simulink model "SS_angulo_pos_planta_CLOSELOOP_simulink"  (R2023b)
settings: Solver=VariableStepAuto  StartTime=0.0  StopTime=15  RelTol=1e-6
values from neighbouring files (symbols this model uses):
  Planta = ss([0 0 1 0;0 0 0 1;0 0 -11.48 0;0 -35.39 0 -0.01639],[0;-0.3736;0.2846;-0.8948],[1 0 0 0;0 1 0 0],0)    [Script_generador.m]
undefined symbols (not defined in the file or in its folder): SS_An, SS_Po
settings Model: Creator=natih  LastModifiedBy=jmarin

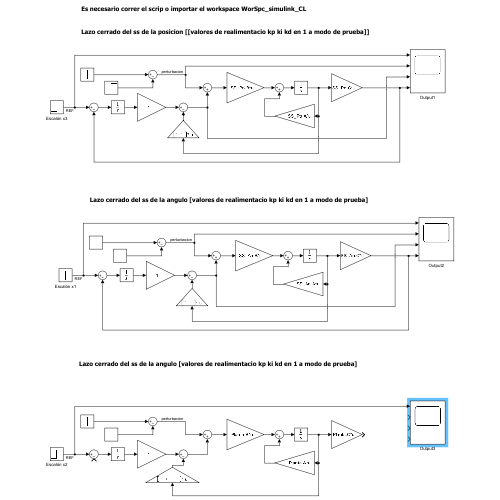
[thumbnail: Simulink's stored preview of the top-level diagram]
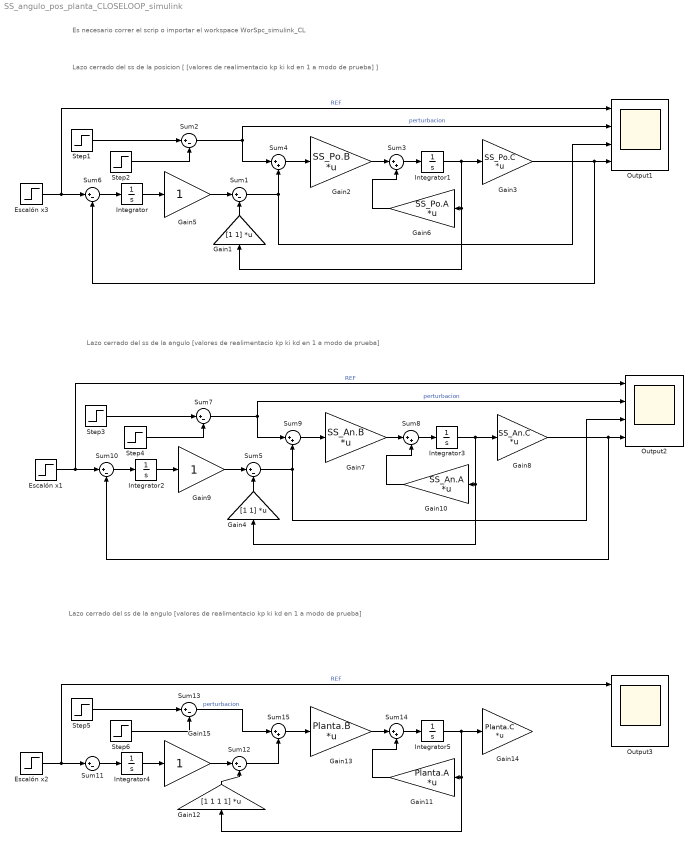
== system SS_angulo_pos_planta_CLOSELOOP_simulink ==
  note: Lazo cerrado del ss de la posicion [ [valores de realimentacio kp ki kd en 1 a modo de prueba] ]
  note: Lazo cerrado del ss de la angulo [valores de realimentacio kp ki kd en 1 a modo de prueba]
  note: Es necesario correr el scrip o importar el workspace WorSpc_simulink_CL
  note: Lazo cerrado del ss de la angulo [valores de realimentacio kp ki kd en 1 a modo de prueba]
  Escalón x1 : Step  Time=0.5  SampleTime=0
  Escalón x2 : Step  Time=0.5  SampleTime=0
  Escalón x3 : Step  Time=0.5  SampleTime=0
  Gain1 : Gain  Gain=[1 1]  Multiplication=Matrix(K*u)
  Gain10 : Gain  Gain=SS_An.A  Multiplication=Matrix(K*u)
  Gain11 : Gain  Gain=Planta.A  Multiplication=Matrix(K*u)
  Gain12 : Gain  Gain=[1 1 1 1]  Multiplication=Matrix(K*u)
  Gain13 : Gain  Gain=Planta.B  Multiplication=Matrix(K*u)
  Gain14 : Gain  Gain=Planta.C  Multiplication=Matrix(K*u)
  Gain15 : Gain
  Gain2 : Gain  Gain=SS_Po.B  Multiplication=Matrix(K*u)
  Gain3 : Gain  Gain=SS_Po.C  Multiplication=Matrix(K*u)
  Gain4 : Gain  Gain=[1 1]  Multiplication=Matrix(K*u)
  Gain5 : Gain
  Gain6 : Gain  Gain=SS_Po.A  Multiplication=Matrix(K*u)
  Gain7 : Gain  Gain=SS_An.B  Multiplication=Matrix(K*u)
  Gain8 : Gain  Gain=SS_An.C  Multiplication=Matrix(K*u)
  Gain9 : Gain
  Integrator{,1..5} (6 alike) : Integrator
  Output1 : Scope  NumInputPorts=4
  Output2 : Scope  NumInputPorts=4
  Output3 : Scope  NumInputPorts=4
  Step1 : Step  Time=6  After=0.3  SampleTime=0
  Step2 : Step  Time=11  After=0.3  SampleTime=0
  Step3 : Step  Time=6  After=0.3  SampleTime=0
  Step4 : Step  Time=11  After=0.3  SampleTime=0
  Step5 : Step  Time=6  After=0.3  SampleTime=0
  Step6 : Step  Time=11  After=0.3  SampleTime=0
  Sum{1..2,5..7,10..13} (9 alike) : Sum  Inputs=|+-
  Sum{3..4,8..9,14..15} (6 alike) : Sum  Inputs=|++
  wires:
  Step1/1 -> Sum2/1
  Escalón x3/1 -> Output1/1, Sum6/1  "REF"
  Step2/1 -> Sum2/2
  Sum6/1 -> Integrator/1
  Integrator/1 -> Gain5/1
  Gain5/1 -> Sum1/1
  Gain2/1 -> Sum3/1
  Sum3/1 -> Integrator1/1
  Integrator1/1 -> Gain1/1, Gain6/1, Gain3/1
  Gain3/1 -> Sum6/2, Output1/4
  Gain1/1 -> Sum1/2
  Gain6/1 -> Sum3/2
  Sum2/1 -> Sum4/1, Output1/2  "perturbacion"
  Sum1/1 -> Sum4/2, Output1/3
  Sum4/1 -> Gain2/1
  Gain8/1 -> Sum10/2, Output2/4
  Integrator3/1 -> Gain4/1, Gain10/1, Gain8/1
  Gain4/1 -> Sum5/2
  Integrator2/1 -> Gain9/1
  Sum7/1 -> Sum9/1, Output2/2  "perturbacion"
  Sum10/1 -> Integrator2/1
  Step3/1 -> Sum7/1
  Gain9/1 -> Sum5/1
  Gain7/1 -> Sum8/1
  Sum8/1 -> Integrator3/1
  Gain10/1 -> Sum8/2
  Sum5/1 -> Sum9/2, Output2/3
  Sum9/1 -> Gain7/1
  Escalón x1/1 -> Output2/1, Sum10/1  "REF"
  Step4/1 -> Sum7/2
  Step6/1 -> Sum13/2
  Escalón x2/1 -> Output3/1, Sum11/1  "REF"
  Sum15/1 -> Gain13/1
  Sum12/1 -> Sum15/2
  Integrator5/1 -> Gain12/1, Gain11/1, Gain14/1
  Sum11/1 -> Integrator4/1
  Gain13/1 -> Sum14/1
  Step5/1 -> Sum13/1
  Gain12/1 -> Sum12/2
  Sum13/1 -> Sum15/1  "perturbacion"
  Integrator4/1 -> Gain15/1
  Sum14/1 -> Integrator5/1
  Gain15/1 -> Sum12/1
  Gain11/1 -> Sum14/2
